simulink model "theta_vp"  (R2024a)
settings: Solver=VariableStepAuto  StartTime=0.0  StopTime=10  RelTol=1e-3
values from neighbouring files (symbols this model uses):
  den_thetaVP = [Jeq*Lm / (Kt*N), Jeq*Rm / (Kt*N), Kb*N, 0]    [preprocess.m]
  num_thetaVp = [-1]    [preprocess.m]
settings Model: Creator=dunni  LastModifiedBy=dunni

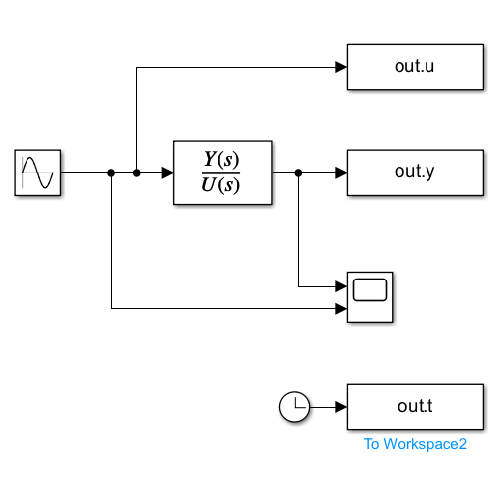
[thumbnail: Simulink's stored preview of the top-level diagram]
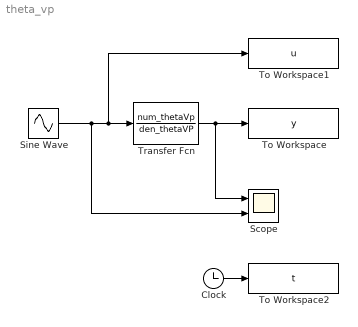
== system theta_vp ==
  Clock : Clock
  Scope : Scope  NumInputPorts=2
  Sine Wave : Sin  Frequency=2*pi  SampleTime=0
  To Workspace : ToWorkspace  VariableName=y  SampleTime=-1
  To Workspace1 : ToWorkspace  VariableName=u  SampleTime=-1
  To Workspace2 : ToWorkspace  VariableName=t  SampleTime=-1
  Transfer Fcn : TransferFcn  Numerator=num_thetaVp  Denominator=den_thetaVP
  wires:
  Sine Wave/1 -> Scope/2, To Workspace1/1, Transfer Fcn/1
  Transfer Fcn/1 -> Scope/1, To Workspace/1
  Clock/1 -> To Workspace2/1
